simulink model "MIL_Fuel_Filter_Model"  (R2019a)
settings: Solver=FixedStepDiscrete  StartTime=0.0  StopTime=500  FixedStep=0.01  RelTol=1e-3
undefined symbols (not defined in the file or in its folder): Constant_0, Constant_1, Constant_100, Constant_5, Constant_50, Error_code_101, Error_code_102, resistance_constant, sigbuilder_block
libraries: simulink x3
settings Model: DataDictionary=Fuel_filter_1.sldd  OrderedModelArguments=off  Creator=Akshay  LastModifiedBy=Akshay
settings OptimizationCC: DefaultParameterBehavior=Inlined  EnhancedBackFolding=on  PassReuseOutputArgsAs=Individual arguments  OptimizeBlockOrder=speed  DifferentSizesBufferReuse=on  OptimizationCustomize=off
settings DebuggingCC: ParameterOverflowMsg=none  ParameterTunabilityLossMsg=error
settings SFSimCC: MATLABDynamicMemAlloc=off
settings RTWCC: SystemTargetFile=ert.tlc  GenCodeOnly=on  TemplateMakefile=ert_default_tmf  GenerateReport=on  IncludeHyperlinkInReport=on  LaunchReport=on  GenerateTraceInfo=on  GenerateTraceReport=on  GenerateTraceReportSl=on  GenerateTraceReportSf=on  GenerateTraceReportEml=on
settings CodeAppCC: ForceParamTrailComments=on  IgnoreCustomStorageClasses=off  OperatorAnnotations=on  SimulinkDataObjDesc=on  SFDataObjDesc=on  InsertBlockDesc=on
settings ERTTargetCC: TargetLangStandard=C99 (ISO)  GenerateSampleERTMain=on  InlinedParameterPlacement=NonHierarchical  ERTCustomFileTemplate=example_file_process.tlc
settings ConfigComp: CovEnable=on  RecordCoverage=on  CovMetricSettings=dcmwe  CovModelRefEnable=on  DVMaxProcessTime=1000  DVParametersUseConfig=on  DVModelCoverageObjectives=MCDC  DVTestSuiteOptimization=Auto  DVDetectOutOfBounds=on  DVDetectInfNaN=on  DVDetectSubnormal=on  DVDesignMinMaxCheck=on  DVProvingStrategy=ProveWithViolationDetection  DVSaveReport=on  DVReportPDFFormat=on  DVRebuildModelRepresentation=Always

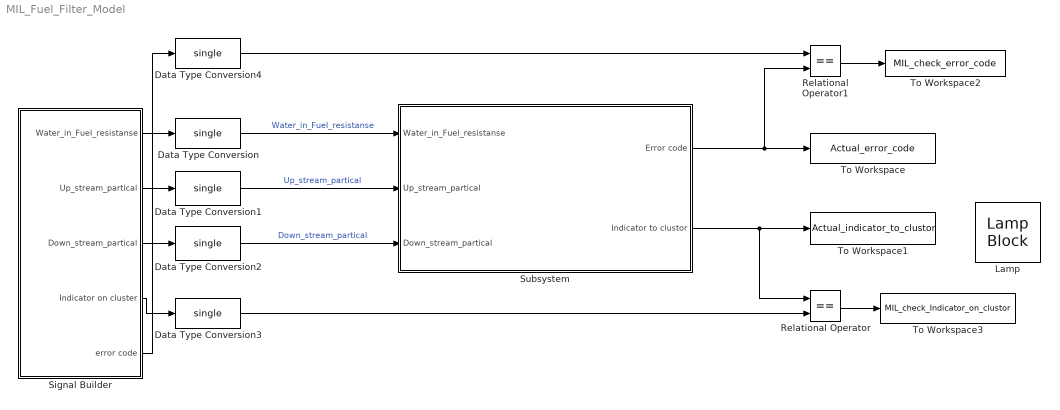
== system MIL_Fuel_Filter_Model ==
  Data Type Conversion{,1..4} (5 alike) : DataTypeConversion  OutDataTypeStr=single
  Lamp : LampBlock
  Relational Operator : RelationalOperator  Operator===  OutDataTypeStr=boolean  RndMeth=Simplest
  Relational Operator1 : RelationalOperator  Operator===  OutDataTypeStr=boolean  RndMeth=Simplest
  Signal Builder : Subsystem  Tag=STV Subsys  LoadFcn=sigbuilder_block('load');  StartFcn=sigbuilder_block('start');  StopFcn=sigbuilder_block('stop');  ClipboardFcn=sigbuilder_block('clipboard');  mask(Sigbuilder block){tuvar=[0:10]}
      mask help: Simulink:masks:SigbuilderBlock_MD
      mask init:
      | if ~strcmp(get_param(bdroot(gcbh),'SimulationStatus'),'stopped') tuvar = sigbuilder_block('maskInit'); end
      settings: CopyFcn=sigbuilder_block('copy');  DeleteFcn=sigbuilder_block('delete');  ModelCloseFcn=sigbuilder_block('modelClose');  PreSaveFcn=sigbuilder_block('preSave');  PauseFcn=sigbuilder_block('pause');  ContinueFcn=sigbuilder_block('continue');  NameChangeFcn=sigbuilder_block('namechange');  OpenFcn=sigbuilder_block('open',[437.6 199.2 550.4 400 ]);  CloseFcn=sigbuilder_block('close');
      mask Display: plot(0, 0, 100, 100,[2, 2, 32, 32, 2], [68, 8, 8, 68, 68],[32, 2], [38, 38], [32, 19, 2],[53, 60, 44], [32, 17, 17, 2],[16, 16, 31, 31]);txt = getActiveGroup(gcbh);text(2, 100, txt,'verticalAlignment', 'top');
  Subsystem : Subsystem  TreatAsAtomicUnit=on
  To Workspace : ToWorkspace  VariableName=Actual_error_code  SaveFormat=Timeseries  SampleTime=-1
  To Workspace1 : ToWorkspace  VariableName=Actual_indicator_to_clustor  SaveFormat=Timeseries  SampleTime=-1
  To Workspace2 : ToWorkspace  VariableName=MIL_check_error_code  SaveFormat=Timeseries  SampleTime=-1
  To Workspace3 : ToWorkspace  VariableName=MIL_check_Indicator_on_clustor  SaveFormat=Timeseries  SampleTime=-1
  wires:
  Subsystem/2(Indicator to clustor) -> Relational Operator/1, To Workspace1/1
  Relational Operator/1 -> To Workspace3/1
  Signal Builder/4(Indicator on cluster) -> Data Type Conversion3/1
  Relational Operator1/1 -> To Workspace2/1
  Signal Builder/5(error code) -> Data Type Conversion4/1
  Data Type Conversion3/1 -> Relational Operator/2
  Data Type Conversion4/1 -> Relational Operator1/1
  Signal Builder/2(Up_stream_partical) -> Data Type Conversion1/1
  Signal Builder/3(Down_stream_partical) -> Data Type Conversion2/1
  Signal Builder/1(Water_in_Fuel_resistanse) -> Data Type Conversion/1
  Data Type Conversion/1 -> Subsystem/1(Water_in_Fuel_resistanse)  "Water_in_Fuel_resistanse"
  Data Type Conversion1/1 -> Subsystem/2(Up_stream_partical)  "Up_stream_partical"
  Data Type Conversion2/1 -> Subsystem/3(Down_stream_partical)  "Down_stream_partical"
  Subsystem/1(Error code) -> To Workspace/1, Relational Operator1/2

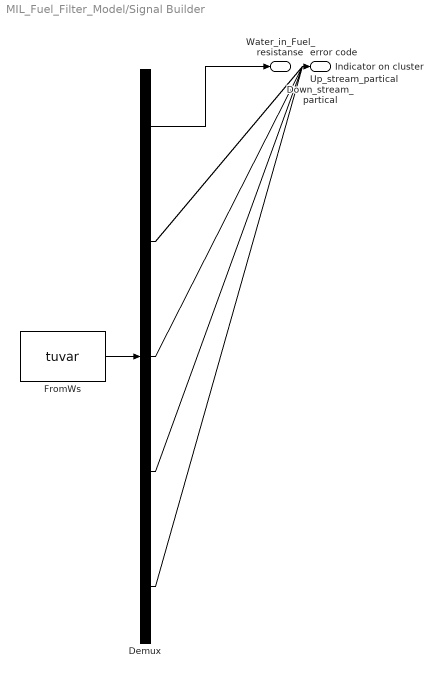
== system MIL_Fuel_Filter_Model/Signal Builder ==
  Demux : Demux  Tag=STV Demux  Outputs=5
  FromWs : FromWorkspace  Tag=STV FromWs  VariableName=tuvar  SampleTime=0
      SigBuilderData=|
      | common.afterFinalStr = 'Extrapolate'
      | common.sampleTime = 0
      | dataSet.timeRange = [0 2.27]
      | dataSet.name = 'Sheet1'
      | sbobj.Name = 'Signal Builder'
      | sbobj.Groups.Name = 'Sheet1'
      | sbobj.Groups.Signals(1).Name = 'Water_in_Fuel_resistanse'
      | sbobj.Groups.Signals(1).XData = [0 0.01 0.02 0.03 0.04 0.05 0.06 0.07 0.08 0.09 0.1 0.11 0.12 0.13 0.14 0.15 0.16 0.17 0.18 0.19 0.2 0.21 0.22 0.23 0.24 0.25 0.26 0.27 0.28 0.29 0.3 0.31 0.32 0.33 0.34 0.35 0.36 0.37 0.38 0.39 0.4 0.41 0.42 0.43 0.44 0.45 0.46 0.47 0.48 0.49 0.5 0.51 0.52 0.53 0.54 0.55 0.56 0.57 0.58 0.59 0.6 0.61 0.62 0.63 0.64 0.65 0.66 0.67 0.68 0.69 0.7 0.71 0.72 0.73 0.74 0.75 0.76 0.77 0.78 0.79 0.8 0.81 0.82 0.83 0.84 0.85 0.86 0.87 0.88 0.89 0.9 0.91 0.92 0.93 0.94 0.95 0.96 0.97 0.98 0.99 1 1.01 1.02 1.03 1.04 1.05 1.06 1.07 1.08 1.09 1.1 1.11 1.12 1.13 1.14 1.15 1.16 1.17 1.18 1.19 1.2 1.21 1.22 1.23 1.24 1.25 1.26 1.27 1.28 1.29 1.3 1.31 1.32 1.33 1.34 1.35 1.36 1.37 1.38 1.39 1.4 1.41 1.42 1.43 1.44 1.45 1.46 1.47 1.48 1.49 1.5 1.51 1.52 1.53 1.54 1.55 1.56 1.57 1.58 1.59 1.6 1.61 1.62 1.63 1.64 1.65 1.66 1.67 1.68 1.69 1.7 1.71 1.72 1.73 1.74 1.75 1.76 1.77 1.78 1.79 1.8 1.81 1.82 1.83 1.84 1.85 1.86 1.87 1.88 1.89 1.9 1.91 1.92 1.93 1.94 1.95 1.96 1.97 1.98 1.99 2 2.01 2.02 2.03 2.04 2.05 2.06 2.07 2.08 2.09 2.1 2.11 2.12 2.13 2.14 2.15 2.16 2.17 2.18 2.19 2.2 2.21 2.22 2.23 2.24 2.25 2.26 2.27]
      | sbobj.Groups.Signals(1).YData = [1 17 143 184 178 146 137 187 194 200 246 46 87 200 34 53 178 39 169 157 198 143 143 143 143 143 143 143 191 191 191 191 191 191 160 190 190 190 190 190 190 189 300 189 189 189 189 190 191 190 191 190 191 190 189 187 190 200 176 157 135 175 174 185 200 245 198 195 206 205 250 300 267 295 248 285 267 195 190 246 200 245 198 195 206 205 250 300 267 295 248 285 267 195 190 246 200 245 198 195 206 205 250 300 267 295 248 285 267 195 190 246 200 245 198 195 206 205 250 300 267 295 248 285 267 195 190 246 1 17 143 184 178 146 137 187 194 200 246 46 87 200 34 53 178 39 169 157 198 143 143 143 143 143 143 143 191 191 191 191 191 191 160 190 190 190 190 190 190 189 300 189 189 189 189 190 191 190 191 190 191 190 189 187 190 200 176 157 135 175 174 185 1 17 143 184 178 146 137 187 194 198 199 200 233 184 183 198 178 39 169 157 198 143 140 129 130 155 176 143 154 145 136 156 178 198 198 198]
      | sbobj.Groups.Signals(2).Name = 'Up_stream_partical'
      | sbobj.Groups.Signals(2).XData = [0 0.01 0.02 0.03 0.04 0.05 0.06 0.07 0.08 0.09 0.1 0.11 0.12 0.13 0.14 0.15 0.16 0.17 0.18 0.19 0.2 0.21 0.22 0.23 0.24 0.25 0.26 0.27 0.28 0.29 0.3 0.31 0.32 0.33 0.34 0.35 0.36 0.37 0.38 0.39 0.4 0.41 0.42 0.43 0.44 0.45 0.46 0.47 0.48 0.49 0.5 0.51 0.52 0.53 0.54 0.55 0.56 0.57 0.58 0.59 0.6 0.61 0.62 0.63 0.64 0.65 0.66 0.67 0.68 0.69 0.7 0.71 0.72 0.73 0.74 0.75 0.76 0.77 0.78 0.79 0.8 0.81 0.82 0.83 0.84 0.85 0.86 0.87 0.88 0.89 0.9 0.91 0.92 0.93 0.94 0.95 0.96 0.97 0.98 0.99 1 1.01 1.02 1.03 1.04 1.05 1.06 1.07 1.08 1.09 1.1 1.11 1.12 1.13 1.14 1.15 1.16 1.17 1.18 1.19 1.2 1.21 1.22 1.23 1.24 1.25 1.26 1.27 1.28 1.29 1.3 1.31 1.32 1.33 1.34 1.35 1.36 1.37 1.38 1.39 1.4 1.41 1.42 1.43 1.44 1.45 1.46 1.47 1.48 1.49 1.5 1.51 1.52 1.53 1.54 1.55 1.56 1.57 1.58 1.59 1.6 1.61 1.62 1.63 1.64 1.65 1.66 1.67 1.68 1.69 1.7 1.71 1.72 1.73 1.74 1.75 1.76 1.77 1.78 1.79 1.8 1.81 1.82 1.83 1.84 1.85 1.86 1.87 1.88 1.89 1.9 1.91 1.92 1.93 1.94 1.95 1.96 1.97 1.98 1.99 2 2.01 2.02 2.03 2.04 2.05 2.06 2.07 2.08 2.09 2.1 2.11 2.12 2.13 2.14 2.15 2.16 2.17 2.18 2.19 2.2 2.21 2.22 2.23 2.24 2.25 2.26 2.27]
      | sbobj.Groups.Signals(2).YData = [1000000 1000000 1000000 1000000 1000000 1000000 1000000 1000000 1000000 1000000 1000000 1000000 1000000 1000000 1000000 1000000 1000000 1000000 1000000 1000000 1000000 1000000 1000000 1000000 1000000 1000000 1000000 1000000 1000000 1000000 1000000 1000000 1000000 1000000 1000000 1000000 1000000 1000000 1000000 1000000 1000000 1000000 1000000 1000000 1000000 1000000 1000000 1000000 1000000 1000000 1000000 1000000 1000000 1000000 1000000 1000000 1000000 1000000 1000000 1000000 1000000 1000000 1000000 1000000 1000000 1000000 1000000 1000000 1000000 1000000 1000000 1000000 1000000 1000000 1000000 1000000 1000000 1000000 1000000 1000000 1000000 1000000 1000000 1000000 1000000 1000000 1000000 1000000 1000000 1000000 1000000 1000000 1000000 1000000 1000000 1000000 1000000 1000000 1000000 1000000 1000000 1000000 1000000 1000000 1000000 1000000 1000000 1000000 1000000 1000000 1000000 1000000 1000000 1000000 1000000 1000000 1000000 1000000 1000000 1000000 1000000 1000000 1000000 1000000 1000000 1000000 1000000 1000000 1000000 1000000 1000000 1000000 1000000 1000000 1000000 1000000 1000000 1000000 1000000 1000000 1000000 1000000 1000000 1000000 1000000 1000000 1000000 1000000 1000000 1000000 1000000 1000000 1000000 1000000 1000000 1000000 1000000 1000000 1000000 1000000 1000000 1000000 1000000 1000000 1000000 1000000 1000000 1000000 1000000 1000000 1000000 1000000 1000000 1000000 1000000 1000000 1000000 1000000 1000000 1000000 1000000 1000000 1000000 1000000 1000000 1000000 1000000 1000000 1000000 1000000 1000000 1000000 1000000 1000000 1000000 1000000 1000000 1000000 1000000 1000000 1000000 1000000 1000000 1000000 1000000 1000000 1000000 1000000 1000000 1000000 1000000 1000000 1000000 1000000 1000000 1000000 1000000 1000000 1000000 1000000 1000000 1000000 1000000 1000000 1000000 1000000 1000000 0]
      | sbobj.Groups.Signals(3).Name = 'Down_stream_partical'
      | sbobj.Groups.Signals(3).XData = [0 0.01 0.02 0.03 0.04 0.05 0.06 0.07 0.08 0.09 0.1 0.11 0.12 0.13 0.14 0.15 0.16 0.17 0.18 0.19 0.2 0.21 0.22 0.23 0.24 0.25 0.26 0.27 0.28 0.29 0.3 0.31 0.32 0.33 0.34 0.35 0.36 0.37 0.38 0.39 0.4 0.41 0.42 0.43 0.44 0.45 0.46 0.47 0.48 0.49 0.5 0.51 0.52 0.53 0.54 0.55 0.56 0.57 0.58 0.59 0.6 0.61 0.62 0.63 0.64 0.65 0.66 0.67 0.68 0.69 0.7 0.71 0.72 0.73 0.74 0.75 0.76 0.77 0.78 0.79 0.8 0.81 0.82 0.83 0.84 0.85 0.86 0.87 0.88 0.89 0.9 0.91 0.92 0.93 0.94 0.95 0.96 0.97 0.98 0.99 1 1.01 1.02 1.03 1.04 1.05 1.06 1.07 1.08 1.09 1.1 1.11 1.12 1.13 1.14 1.15 1.16 1.17 1.18 1.19 1.2 1.21 1.22 1.23 1.24 1.25 1.26 1.27 1.28 1.29 1.3 1.31 1.32 1.33 1.34 1.35 1.36 1.37 1.38 1.39 1.4 1.41 1.42 1.43 1.44 1.45 1.46 1.47 1.48 1.49 1.5 1.51 1.52 1.53 1.54 1.55 1.56 1.57 1.58 1.59 1.6 1.61 1.62 1.63 1.64 1.65 1.66 1.67 1.68 1.69 1.7 1.71 1.72 1.73 1.74 1.75 1.76 1.77 1.78 1.79 1.8 1.81 1.82 1.83 1.84 1.85 1.86 1.87 1.88 1.89 1.9 1.91 1.92 1.93 1.94 1.95 1.96 1.97 1.98 1.99 2 2.01 2.02 2.03 2.04 2.05 2.06 2.07 2.08 2.09 2.1 2.11 2.12 2.13 2.14 2.15 2.16 2.17 2.18 2.19 2.2 2.21 2.22 2.23 2.24 2.25 2.26 2.27]
      | sbobj.Groups.Signals(3).YData = [5000 13000 16000 19000 27000 38000 41000 46000 49000 5000 13000 16000 19000 27000 38000 41000 46000 49000 46000 49000 46000 41000 46000 49000 5000 13000 16000 19000 27000 5000 13000 16000 19000 27000 38000 41000 46000 49000 13000 16000 19000 27000 5000 13000 16000 19000 46000 49000 13000 16000 19000 27000 5000 5000 13000 16000 19000 27000 38000 41000 46000 49000 13000 13000 50000 55000 70000 65000 86000 74000 86000 96000 49000 30000 29000 51000 52000 49000 51000 52000 56000 59000 60000 61000 46000 53000 53000 53000 53000 53000 53000 53000 49000 49000 49000 49000 49000 49000 52000 50000 50000 50000 50000 50000 50000 49000 56000 51000 51000 51000 51000 50000 49000 50000 49000 50000 49000 50000 51000 53000 50000 44000 52000 56000 57000 58000 65000 67000 50000 55000 70000 65000 86000 74000 86000 96000 49000 30000 29000 51000 52000 49000 51000 52000 56000 59000 60000 61000 46000 53000 53000 53000 53000 53000 53000 53000 49000 49000 49000 49000 49000 49000 52000 50000 50000 50000 50000 50000 50000 49000 56000 51000 51000 51000 51000 50000 49000 50000 49000 50000 49000 50000 51000 53000 50000 44000 52000 56000 57000 58000 65000 67000 50000 55000 70000 65000 86000 74000 86000 96000 60000 56000 57000 58000 52000 57000 58000 52000 56000 59000 60000 61000 56000 53000 53000 53000 53000 53000 53000 53000 49000 48000 47000 48000 49000 49000 0 0]
      | sbobj.Groups.Signals(4).Name = 'Indicator on cluster'
      | sbobj.Groups.Signals(4).XData = [0 0.01 0.02 0.03 0.04 0.05 0.06 0.07 0.08 0.09 0.1 0.11 0.12 0.13 0.14 0.15 0.16 0.17 0.18 0.19 0.2 0.21 0.22 0.23 0.24 0.25 0.26 0.27 0.28 0.29 0.3 0.31 0.32 0.33 0.34 0.35 0.36 0.37 0.38 0.39 0.4 0.41 0.42 0.43 0.44 0.45 0.46 0.47 0.48 0.49 0.5 0.51 0.52 0.53 0.54 0.55 0.56 0.57 0.58 0.59 0.6 0.61 0.62 0.63 0.64 0.65 0.66 0.67 0.68 0.69 0.7 0.71 0.72 0.73 0.74 0.75 0.76 0.77 0.78 0.79 0.8 0.81 0.82 0.83 0.84 0.85 0.86 0.87 0.88 0.89 0.9 0.91 0.92 0.93 0.94 0.95 0.96 0.97 0.98 0.99 1 1.01 1.02 1.03 1.04 1.05 1.06 1.07 1.08 1.09 1.1 1.11 1.12 1.13 1.14 1.15 1.16 1.17 1.18 1.19 1.2 1.21 1.22 1.23 1.24 1.25 1.26 1.27 1.28 1.29 1.3 1.31 1.32 1.33 1.34 1.35 1.36 1.37 1.38 1.39 1.4 1.41 1.42 1.43 1.44 1.45 1.46 1.47 1.48 1.49 1.5 1.51 1.52 1.53 1.54 1.55 1.56 1.57 1.58 1.59 1.6 1.61 1.62 1.63 1.64 1.65 1.66 1.67 1.68 1.69 1.7 1.71 1.72 1.73 1.74 1.75 1.76 1.77 1.78 1.79 1.8 1.81 1.82 1.83 1.84 1.85 1.86 1.87 1.88 1.89 1.9 1.91 1.92 1.93 1.94 1.95 1.96 1.97 1.98 1.99 2 2.01 2.02 2.03 2.04 2.05 2.06 2.07 2.08 2.09 2.1 2.11 2.12 2.13 2.14 2.15 2.16 2.17 2.18 2.19 2.2 2.21 2.22 2.23 2.24 2.25 2.26 2.27]
      | sbobj.Groups.Signals(4).YData = [0 0 0 0 0 1 1 1 0 0 0 0 0 0 0 0 0 0 0 1 0 0 0 0 0 0 1 1 0 0 0 0 0 0 0 0 0 0 0 1 1 1 0 0 0 0 0 1 0 0 0 0 0 0 0 0 0 0 0 0 0 0 0 1 0 0 0 0 0 1 1 1 0 0 0 0 0 0 0 0 0 0 0 1 0 0 0 0 0 0 1 1 0 0 0 0 0 0 0 0 0 0 0 1 1 1 0 0 0 0 0 1 0 0 0 0 0 0 0 0 0 0 0 0 0 0 0 1 0 0 0 0 0 1 1 1 0 0 0 0 0 0 0 0 0 0 0 1 0 0 0 0 0 0 1 1 0 0 0 0 0 0 0 0 0 0 0 1 1 1 0 0 0 0 0 1 0 0 0 0 0 0 0 0 0 0 0 0 0 0 0 1 0 0 0 0 0 1 1 1 1 1 1 1 1 1 1 1 1 1 1 1 1 1 1 1 1 1 1 1 1 1 1 1 1 0 0 0]
      | sbobj.Groups.Signals(5).Name = 'error code'
      | sbobj.Groups.Signals(5).XData = [0 0.01 0.02 0.03 0.04 0.05 0.06 0.07 0.08 0.09 0.1 0.11 0.12 0.13 0.14 0.15 0.16 0.17 0.18 0.19 0.2 0.21 0.22 0.23 0.24 0.25 0.26 0.27 0.28 0.29 0.3 0.31 0.32 0.33 0.34 0.35 0.36 0.37 0.38 0.39 0.4 0.41 0.42 0.43 0.44 0.45 0.46 0.47 0.48 0.49 0.5 0.51 0.52 0.53 0.54 0.55 0.56 0.57 0.58 0.59 0.6 0.61 0.62 0.63 0.64 0.65 0.66 0.67 0.68 0.69 0.7 0.71 0.72 0.73 0.74 0.75 0.76 0.77 0.78 0.79 0.8 0.81 0.82 0.83 0.84 0.85 0.86 0.87 0.88 0.89 0.9 0.91 0.92 0.93 0.94 0.95 0.96 0.97 0.98 0.99 1 1.01 1.02 1.03 1.04 1.05 1.06 1.07 1.08 1.09 1.1 1.11 1.12 1.13 1.14 1.15 1.16 1.17 1.18 1.19 1.2 1.21 1.22 1.23 1.24 1.25 1.26 1.27 1.28 1.29 1.3 1.31 1.32 1.33 1.34 1.35 1.36 1.37 1.38 1.39 1.4 1.41 1.42 1.43 1.44 1.45 1.46 1.47 1.48 1.49 1.5 1.51 1.52 1.53 1.54 1.55 1.56 1.57 1.58 1.59 1.6 1.61 1.62 1.63 1.64 1.65 1.66 1.67 1.68 1.69 1.7 1.71 1.72 1.73 1.74 1.75 1.76 1.77 1.78 1.79 1.8 1.81 1.82 1.83 1.84 1.85 1.86 1.87 1.88 1.89 1.9 1.91 1.92 1.93 1.94 1.95 1.96 1.97 1.98 1.99 2 2.01 2.02 2.03 2.04 2.05 2.06 2.07 2.08 2.09 2.1 2.11 2.12 2.13 2.14 2.15 2.16 2.17 2.18 2.19 2.2 2.21 2.22 2.23 2.24 2.25 2.26 2.27]
      | sbobj.Groups.Signals(5).YData = [0 0 0 0 0 101 101 101 0 0 0 0 0 0 0 0 0 0 0 101 0 0 0 0 0 0 101 101 0 0 0 0 0 0 0 0 0 0 0 101 101 101 0 0 0 0 0 101 0 0 0 0 0 0 0 0 0 0 0 0 0 0 0 101 0 0 0 0 0 102 102 102 0 0 0 0 0 0 0 0 0 0 0 102 0 0 0 0 0 0 102 102 0 0 0 0 0 0 0 0 0 0 0 101 101 101 0 0 0 0 0 101 0 0 0 0 0 0 0 0 0 0 0 0 0 0 0 101 0 0 0 0 0 101 101 101 0 0 0 0 0 0 0 0 0 0 0 101 0 0 0 0 0 0 101 101 0 0 0 0 0 0 0 0 0 0 0 101 101 101 0 0 0 0 0 101 0 0 0 0 0 0 0 0 0 0 0 0 0 0 0 101 0 0 0 0 0 101 101 101 102 102 102 102 102 102 102 102 102 102 101 101 102 102 102 102 102 102 101 101 101 101 101 101 101 0 0 0]
      | sbobj.Groups.TimeRange = [0 2.27]
  Water_in_Fuel_resistanse : Outport  Tag=STV Outport
  Up_stream_partical : Outport  Tag=STV Outport  Port=2
  Down_stream_partical : Outport  Tag=STV Outport  Port=3
  Indicator on cluster : Outport  Tag=STV Outport  Port=4
  error code : Outport  Tag=STV Outport  Port=5
  wires:
  Demux/1 -> Water_in_Fuel_resistanse/1
  FromWs/1 -> Demux/1
  Demux/2 -> Up_stream_partical/1
  Demux/3 -> Down_stream_partical/1
  Demux/4 -> Indicator on cluster/1
  Demux/5 -> error code/1

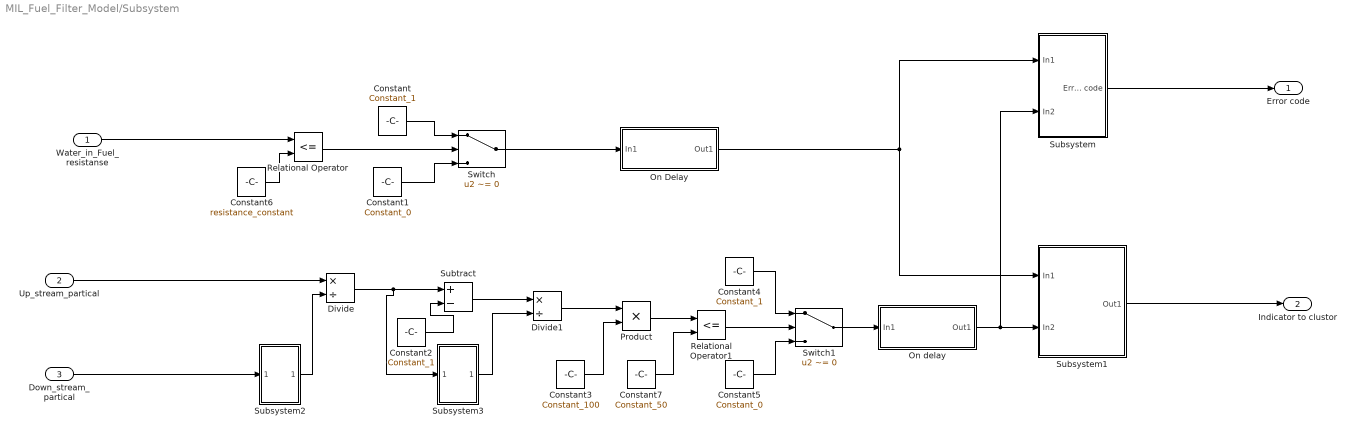
== system MIL_Fuel_Filter_Model/Subsystem ==
  Water_in_Fuel_resistanse : Inport  OutDataTypeStr=single
  Up_stream_partical : Inport  Port=2  OutDataTypeStr=single
  Down_stream_partical : Inport  Port=3  OutDataTypeStr=single
  Constant : Constant  Value=Constant_1  OutDataTypeStr=single
  Constant1 : Constant  Value=Constant_0  OutDataTypeStr=single
  Constant2 : Constant  Value=Constant_1  OutDataTypeStr=single
  Constant3 : Constant  Value=Constant_100  OutDataTypeStr=single
  Constant4 : Constant  Value=Constant_1  OutDataTypeStr=single
  Constant5 : Constant  Value=Constant_0  OutDataTypeStr=single
  Constant6 : Constant  Value=resistance_constant  OutDataTypeStr=single
  Constant7 : Constant  Value=Constant_50  OutDataTypeStr=single
  Divide : Product  Inputs=*/  OutDataTypeStr=single  RndMeth=Ceiling
  Divide1 : Product  Inputs=*/  OutDataTypeStr=single  RndMeth=Ceiling
  On Delay : Subsystem
  On delay : Subsystem
  Product : Product  OutDataTypeStr=single  RndMeth=Ceiling
  Relational Operator : RelationalOperator  Operator=<=  OutDataTypeStr=boolean  RndMeth=Simplest
  Relational Operator1 : RelationalOperator  Operator=<=  OutDataTypeStr=boolean  RndMeth=Simplest
  Subsystem : Subsystem
  Subsystem1 : Subsystem
  Subsystem2 : Subsystem
  Subsystem3 : Subsystem
  Subtract : Sum  Inputs=+-  AccumDataTypeStr=single  OutDataTypeStr=single  RndMeth=Ceiling
  Switch : Switch  Criteria=u2 ~= 0  OutDataTypeStr=single
  Switch1 : Switch  Criteria=u2 ~= 0  OutDataTypeStr=single
  Error code : Outport  OutDataTypeStr=single
  Indicator to clustor : Outport  Port=2  OutDataTypeStr=boolean
  wires:
  Water_in_Fuel_resistanse/1 -> Relational Operator/1
  Relational Operator/1 -> Switch/2
  Constant/1 -> Switch/1
  Constant1/1 -> Switch/3
  Up_stream_partical/1 -> Divide/1
  Divide/1 -> Subsystem3/1(In1), Subtract/1
  Constant2/1 -> Subtract/2
  Subtract/1 -> Divide1/1
  Divide1/1 -> Product/1
  Constant3/1 -> Product/2
  Product/1 -> Relational Operator1/1
  Relational Operator1/1 -> Switch1/2
  Constant4/1 -> Switch1/1
  Constant5/1 -> Switch1/3
  Switch1/1 -> On delay/1(In1)
  Subsystem/1(Error code) -> Error code/1
  Switch/1 -> On Delay/1(In1)
  Subsystem1/1(Out1) -> Indicator to clustor/1
  Constant6/1 -> Relational Operator/2
  Constant7/1 -> Relational Operator1/2
  On Delay/1(Out1) -> Subsystem1/1(In1), Subsystem/1(In1)
  On delay/1(Out1) -> Subsystem/2(In2), Subsystem1/2(In2)
  Down_stream_partical/1 -> Subsystem2/1(In1)
  Subsystem2/1(Out1) -> Divide/2
  Subsystem3/1(Out1) -> Divide1/2

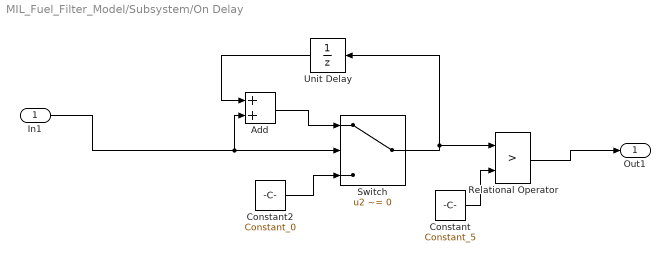
== system MIL_Fuel_Filter_Model/Subsystem/On Delay ==
  In1 : Inport  OutDataTypeStr=single
  Add : Sum  AccumDataTypeStr=single  OutDataTypeStr=single
  Constant : Constant  Value=Constant_5  OutDataTypeStr=single
  Constant2 : Constant  Value=Constant_0  OutDataTypeStr=single
  Relational Operator : RelationalOperator  Operator=>  OutDataTypeStr=boolean  RndMeth=Simplest
  Switch : Switch  Criteria=u2 ~= 0  OutDataTypeStr=single
  Unit Delay : UnitDelay  SampleTime=-1  HasFrameUpgradeWarning=on
  Out1 : Outport  OutDataTypeStr=boolean
  wires:
  Switch/1 -> Unit Delay/1, Relational Operator/1
  In1/1 -> Add/2, Switch/2
  Constant2/1 -> Switch/3
  Add/1 -> Switch/1
  Unit Delay/1 -> Add/1
  Relational Operator/1 -> Out1/1
  Constant/1 -> Relational Operator/2

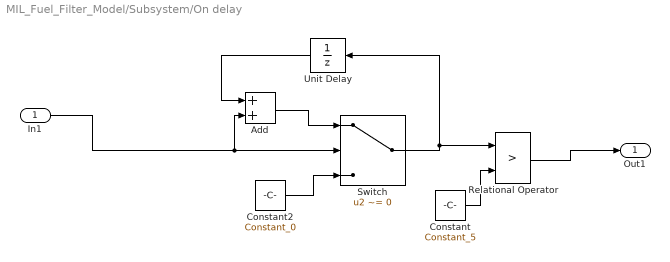
== system MIL_Fuel_Filter_Model/Subsystem/On delay ==
  In1 : Inport  OutDataTypeStr=single
  Add : Sum  AccumDataTypeStr=single  OutDataTypeStr=single
  Constant : Constant  Value=Constant_5  OutDataTypeStr=single
  Constant2 : Constant  Value=Constant_0  OutDataTypeStr=single
  Relational Operator : RelationalOperator  Operator=>  OutDataTypeStr=boolean  RndMeth=Simplest
  Switch : Switch  Criteria=u2 ~= 0  OutDataTypeStr=single
  Unit Delay : UnitDelay  SampleTime=-1  HasFrameUpgradeWarning=on
  Out1 : Outport  OutDataTypeStr=boolean
  wires:
  Constant/1 -> Relational Operator/2
  Relational Operator/1 -> Out1/1
  Unit Delay/1 -> Add/1
  Add/1 -> Switch/1
  Constant2/1 -> Switch/3
  In1/1 -> Switch/2, Add/2
  Switch/1 -> Relational Operator/1, Unit Delay/1

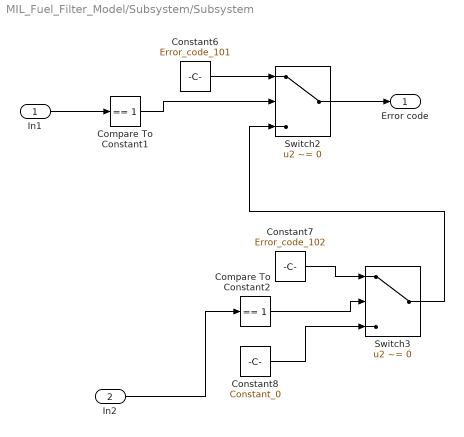
== system MIL_Fuel_Filter_Model/Subsystem/Subsystem ==
  In1 : Inport  OutDataTypeStr=boolean
  In2 : Inport  Port=2  OutDataTypeStr=boolean
  Compare To Constant1 : simulink/Logic and Bit Operations/Compare To Constant  relop===  const=1  OutDataTypeStr=boolean
  Compare To Constant2 : simulink/Logic and Bit Operations/Compare To Constant  relop===  const=1  OutDataTypeStr=boolean
  Constant6 : Constant  Value=Error_code_101  OutDataTypeStr=int8
  Constant7 : Constant  Value=Error_code_102  OutDataTypeStr=single
  Constant8 : Constant  Value=Constant_0  OutDataTypeStr=single
  Switch2 : Switch  Criteria=u2 ~= 0  OutDataTypeStr=single
  Switch3 : Switch  Criteria=u2 ~= 0  OutDataTypeStr=single
  Error code : Outport  OutDataTypeStr=single
  wires:
  Switch3/1 -> Switch2/3
  Constant7/1 -> Switch3/1
  Switch2/1 -> Error code/1
  In1/1 -> Compare To Constant1/1
  Constant6/1 -> Switch2/1
  In2/1 -> Compare To Constant2/1
  Constant8/1 -> Switch3/3
  Compare To Constant1/1 -> Switch2/2
  Compare To Constant2/1 -> Switch3/2

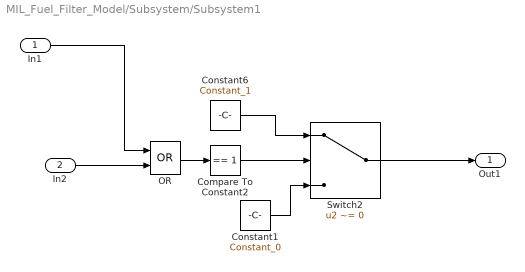
== system MIL_Fuel_Filter_Model/Subsystem/Subsystem1 ==
  In1 : Inport  OutDataTypeStr=boolean
  In2 : Inport  Port=2  OutDataTypeStr=boolean
  Compare To Constant2 : simulink/Logic and Bit Operations/Compare To Constant  relop===  const=1  OutDataTypeStr=boolean
  Constant1 : Constant  Value=Constant_0  OutDataTypeStr=single
  Constant6 : Constant  Value=Constant_1  OutDataTypeStr=single
  OR : Logic  Operator=OR  AllPortsSameDT=off  OutDataTypeStr=boolean
  Switch2 : Switch  Criteria=u2 ~= 0  OutDataTypeStr=boolean
  Out1 : Outport  OutDataTypeStr=boolean
  wires:
  In2/1 -> OR/2
  In1/1 -> OR/1
  Compare To Constant2/1 -> Switch2/2
  Constant6/1 -> Switch2/1
  OR/1 -> Compare To Constant2/1
  Switch2/1 -> Out1/1
  Constant1/1 -> Switch2/3

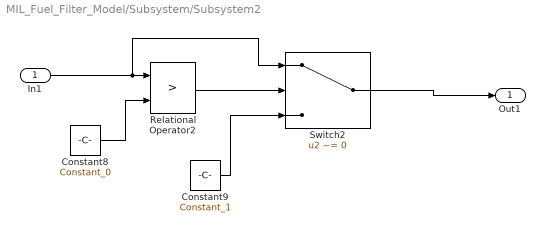
== system MIL_Fuel_Filter_Model/Subsystem/Subsystem2 ==
  In1 : Inport  OutDataTypeStr=single
  Constant8 : Constant  Value=Constant_0  OutDataTypeStr=single
  Constant9 : Constant  Value=Constant_1  OutDataTypeStr=single
  Relational Operator2 : RelationalOperator  Operator=>  OutDataTypeStr=boolean  RndMeth=Simplest
  Switch2 : Switch  Criteria=u2 ~= 0  OutDataTypeStr=single
  Out1 : Outport  OutDataTypeStr=single
  wires:
  Constant8/1 -> Relational Operator2/2
  In1/1 -> Switch2/1, Relational Operator2/1
  Switch2/1 -> Out1/1
  Constant9/1 -> Switch2/3
  Relational Operator2/1 -> Switch2/2

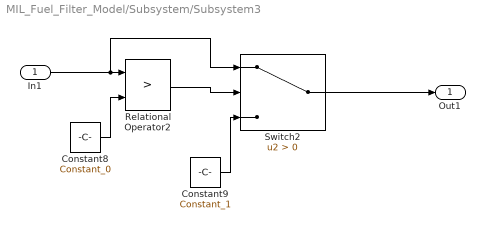
== system MIL_Fuel_Filter_Model/Subsystem/Subsystem3 ==
  In1 : Inport  OutDataTypeStr=single
  Constant8 : Constant  Value=Constant_0  OutDataTypeStr=single
  Constant9 : Constant  Value=Constant_1  OutDataTypeStr=single
  Relational Operator2 : RelationalOperator  Operator=>  OutDataTypeStr=boolean  RndMeth=Simplest
  Switch2 : Switch  Criteria=u2 > Threshold  OutDataTypeStr=single
  Out1 : Outport  OutDataTypeStr=single
  wires:
  Relational Operator2/1 -> Switch2/2
  Constant9/1 -> Switch2/3
  Switch2/1 -> Out1/1
  In1/1 -> Switch2/1, Relational Operator2/1
  Constant8/1 -> Relational Operator2/2
